simulink model "sldemo_varsize_channel_pow_alloc"  (R2019b)
settings: Solver=FixedStepDiscrete  StartTime=0.0  StopTime=10.0  RelTol=1e-3  EnableMultiTasking=on
settings Model: Creator=The MathWorks, Inc.  LastModifiedBy=bhisma
settings DataIOCC: LimitDataPoints=on  SaveFormat=Array
settings OptimizationCC: ExpressionDepthLimit=2147483647  LifeSpan=inf
settings DebuggingCC: SolverPrmCheckMsg=warning  FcnCallInpInsideContextMsg=warning  StateNameClashWarn=warning  SFUnexpectedBacktrackingDiag=warning  SFNoUnconditionalDefaultTransitionDiag=warning  SFExecutionAtInitializationDiag=none  ArithmeticOperatorsInVariantConditions=warning
settings HardwareCC: ProdBitPerPointer=32  ProdBitPerSizeT=32  ProdBitPerPtrDiffT=32  ProdLargestAtomicFloat=None  ProdIntDivRoundTo=Undefined  ProdEndianess=Unspecified  ProdWordSize=32  ProdHWDeviceType=32-bit Generic
settings ModelReferenceCC: PropagateSignalLabelsOutOfModel=off
settings SFSimCC: SimUseLocalCustomCode=off  CustomCodeUndefinedFunction=UseInterfaceOnly
settings RTWCC: RTWUseLocalCustomCode=off
settings CodeAppCC: StateflowObjectComments=on
settings GRTTargetCC: TargetLangStandard=C89/C90 (ANSI)  GeneratePreprocessorConditionals=Disable all  CombineOutputUpdateFcns=off  GRTInterface=on
settings ConfigComp: CovMetricSettings=dw  CovHtmlReporting=on  CovSaveCumulativeToWorkspaceVar=on  CovSaveSingleToWorkspaceVar=on  CovExternalEMLEnable=off

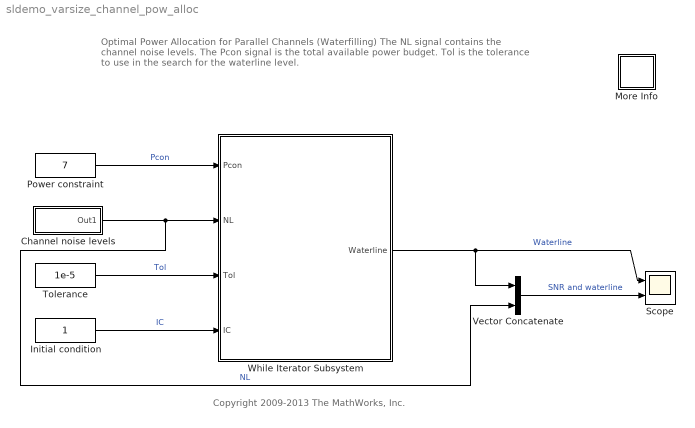
== system sldemo_varsize_channel_pow_alloc ==
  note: Optimal Power Allocation for Parallel Channels (Waterfilling)
      |
      | The NL signal contains the channel noise levels.
      | The Pcon signal is the total available power budget.
      | Tol is the tolerance to use in the search for the waterline level.
  note: Copyright 2009-2013 The MathWorks, Inc.
  Channel noise levels : Subsystem
      mask Display: disp('')
  Initial condition : Constant  OutDataTypeStr=double  SampleTime=1
  More Info : Subsystem
      settings: OpenFcn=showdemo(bdroot(gcb))
      mask Display: disp('?')
  Power constraint : Constant  Value=7  OutDataTypeStr=double  SampleTime=1
  Scope : Scope  NumInputPorts=2
  Tolerance : Constant  Value=1e-5  OutDataTypeStr=double  SampleTime=1
  Vector Concatenate : Concatenate
  While Iterator Subsystem : Subsystem  TreatAsAtomicUnit=on
      mask Display:
      | plot([0 1 1 2 2 3 3 4 4 5 5 6 6 7 0],[0 0 3 3 5 5 2 2 7 7 1 1 0 0 0]);
      | color('red');
      | plot([.5 6.5],[4.5 4.5]);
      | color('blue');
      | plot( [1.5 1.5],[3 4.5])
      | plot( [3.5 3.5],[2 4.5]);
      | plot( [5.5 5.5],[1 4.5]);
      | text( 1.3, 5, 'P1');
      | text( 3.3, 5, 'Pi');
      | text( 5.3, 5, 'Pn');
      | text( 0.3 , 6.3 , 'Pcon = P1+...+Pn');
  wires:
  Power constraint/1 -> While Iterator Subsystem/1(Pcon)  "Pcon"
  Tolerance/1 -> While Iterator Subsystem/3(Tol)  "Tol"
  Initial condition/1 -> While Iterator Subsystem/4(IC)  "IC"
  While Iterator Subsystem/1(Waterline) -> Scope/1, Vector Concatenate/1  "Waterline"
  Vector Concatenate/1 -> Scope/2  "SNR and waterline"
  Channel noise levels/1(Out1) -> While Iterator Subsystem/2(NL), Vector Concatenate/2  "NL"

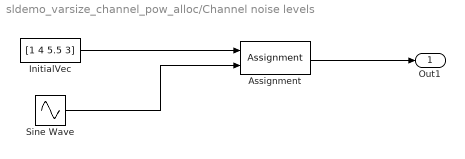
== system sldemo_varsize_channel_pow_alloc/Channel noise levels ==
  Assignment : Assignment  IndexOptions=Index vector (dialog)  Indices=1  OutputSizes=1
  InitialVec : Constant  Value=[1 4 5.5 3]  OutDataTypeStr=double  SampleTime=1
  Sine Wave : Sin  SineType=Sample based  Bias=2  SampleTime=1
  Out1 : Outport  VectorParamsAs1DForOutWhenUnconnected=off
  wires:
  InitialVec/1 -> Assignment/1
  Sine Wave/1 -> Assignment/2
  Assignment/1 -> Out1/1

== system sldemo_varsize_channel_pow_alloc/More Info ==

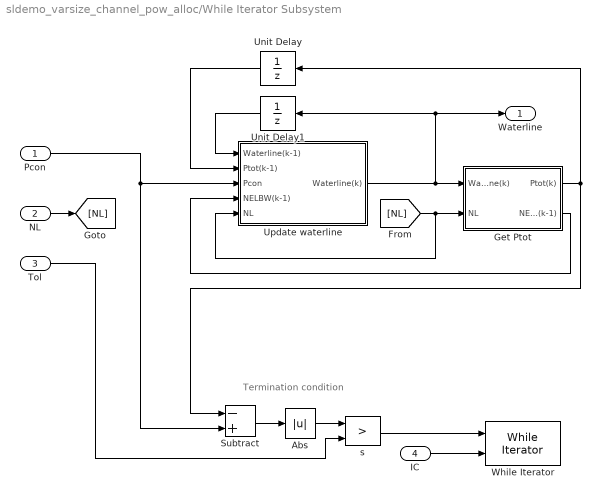
== system sldemo_varsize_channel_pow_alloc/While Iterator Subsystem ==
  note: Termination condition
  Pcon : Inport
  NL : Inport  Port=2
  Tol : Inport  Port=3
  IC : Inport  Port=4
  Abs : Abs
  Get Ptot : Subsystem
      settings: MinAlgLoopOccurrences=on
  Subtract : Sum  Inputs=-+
  Unit Delay : UnitDelay  SampleTime=-1  HasFrameUpgradeWarning=on
  Unit Delay1 : UnitDelay  SampleTime=-1  HasFrameUpgradeWarning=on
  Update waterline : Subsystem
  While Iterator : WhileIterator
  s : RelationalOperator  Operator=>  OutDataTypeStr=boolean  RndMeth=Nearest
  Waterline : Outport  VectorParamsAs1DForOutWhenUnconnected=off
  wires:
  IC/1 -> While Iterator/2
  Update waterline/1(Waterline(k)) -> Unit Delay1/1, Waterline/1, Get Ptot/1(Waterline(k))
  Get Ptot/1(Ptot(k)) -> Unit Delay/1, Subtract/1
  Unit Delay1/1 -> Update waterline/1(Waterline(k-1))
  Unit Delay/1 -> Update waterline/2(Ptot(k-1))
  Pcon/1 -> Update waterline/3(Pcon), Subtract/2
  Subtract/1 -> Abs/1
  Abs/1 -> s/1
  Tol/1 -> s/2
  s/1 -> While Iterator/1
  Get Ptot/2(NELBW(k-1)) -> Update waterline/4(NELBW(k-1))
  [NL] -> Get Ptot/2(NL), Update waterline/5(NL)
  NL/1 -> [NL]

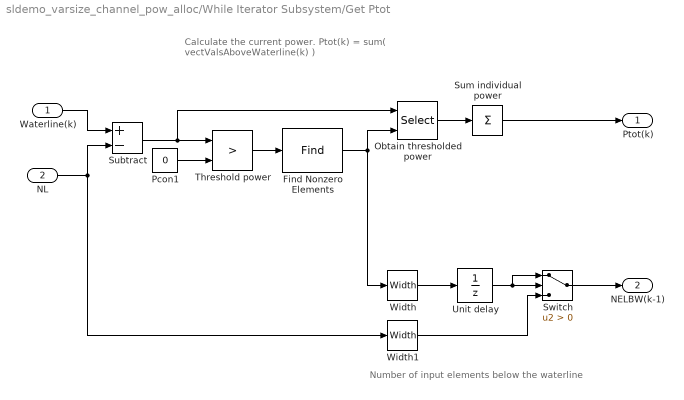
== system sldemo_varsize_channel_pow_alloc/While Iterator Subsystem/Get Ptot ==
  note: Calculate the current power.
      | Ptot(k) = sum( vectValsAboveWaterline(k) )
  note: Number of input elements below the waterline
  Waterline(k) : Inport
  NL : Inport  Port=2
  Find Nonzero Elements : Find  OutDataTypeStr=int8
  Obtain thresholded power : Selector  IndexOptions=Index vector (port)  Indices=[1 3]  OutputSizes=1
  Pcon1 : Constant  Value=0  OutDataTypeStr=double  SampleTime=-1
  Subtract : Sum  Inputs=+-
  Sum individual power : Sum  Inputs=+
  Switch : Switch  Criteria=u2 > Threshold
  Threshold power : RelationalOperator  Operator=>  OutDataTypeStr=boolean  RndMeth=Nearest
  Unit delay : UnitDelay  SampleTime=-1  HasFrameUpgradeWarning=on
  Width : Width
  Width1 : Width
  Ptot(k) : Outport  VectorParamsAs1DForOutWhenUnconnected=off
  NELBW(k-1) : Outport  Port=2  VectorParamsAs1DForOutWhenUnconnected=off
  wires:
  Sum individual power/1 -> Ptot(k)/1
  NL/1 -> Subtract/2, Width1/1
  Waterline(k)/1 -> Subtract/1
  Obtain thresholded power/1 -> Sum individual power/1
  Find Nonzero Elements/1 -> Obtain thresholded power/2, Width/1
  Pcon1/1 -> Threshold power/2
  Subtract/1 -> Obtain thresholded power/1, Threshold power/1
  Threshold power/1 -> Find Nonzero Elements/1
  Width/1 -> Unit delay/1
  Switch/1 -> NELBW(k-1)/1
  Unit delay/1 -> Switch/2, Switch/1
  Width1/1 -> Switch/3

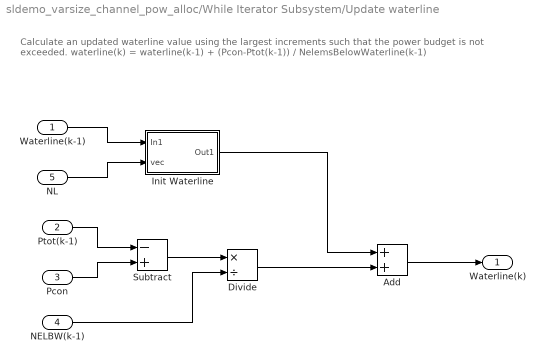
== system sldemo_varsize_channel_pow_alloc/While Iterator Subsystem/Update waterline ==
  note: Calculate an updated waterline value using  the largest increments such that the
      | power budget is not exceeded.
      |
      | waterline(k) = waterline(k-1) + (Pcon-Ptot(k-1)) / NelemsBelowWaterline(k-1)
  Waterline(k-1) : Inport
  Ptot(k-1) : Inport  Port=2
  Pcon : Inport  Port=3
  NELBW(k-1) : Inport  Port=4
  NL : Inport  Port=5
  Add : Sum
  Divide : Product  Inputs=*/
  Init Waterline : Subsystem
  Subtract : Sum  Inputs=-+
  Waterline(k) : Outport  VectorParamsAs1DForOutWhenUnconnected=off
  wires:
  Add/1 -> Waterline(k)/1
  Ptot(k-1)/1 -> Subtract/1
  NELBW(k-1)/1 -> Divide/2
  Subtract/1 -> Divide/1
  Pcon/1 -> Subtract/2
  Divide/1 -> Add/2
  Init Waterline/1(Out1) -> Add/1
  Waterline(k-1)/1 -> Init Waterline/1(In1)
  NL/1 -> Init Waterline/2(vec)

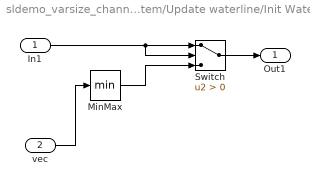
== system sldemo_varsize_channel_pow_alloc/While Iterator Subsystem/Update waterline/Init Waterline ==
  In1 : Inport
  vec : Inport  Port=2
  MinMax : MinMax
  Switch : Switch  Criteria=u2 > Threshold
  Out1 : Outport  VectorParamsAs1DForOutWhenUnconnected=off
  wires:
  In1/1 -> Switch/1, Switch/2
  Switch/1 -> Out1/1
  MinMax/1 -> Switch/3
  vec/1 -> MinMax/1
